simulink model "LoadControltotal2"  (R2013a)
settings: Solver=ode45  StartTime=0.0  StopTime=0.2  RelTol=1e-3
settings Model: Creator=MEHEDI HASSAN  LastModifiedBy=BORAT
settings OptimizationCC: InlineParams=on
settings DebuggingCC: SolverPrmCheckMsg=none  ModelReferenceExtraNoncontSigs=none

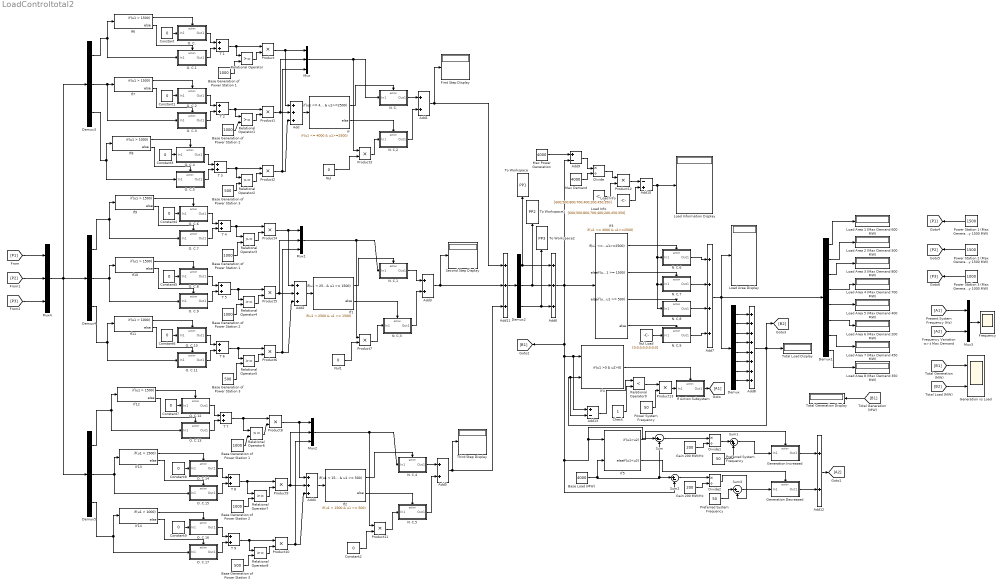
== system LoadControltotal2 ==
  Add{,2,4,6,11} (5 alike) : Sum  Inputs=+++
  Add{1,3,5,12} (4 alike) : Sum
  Add10 : Sum  Inputs=-+
  Add13 : Sum  Inputs=+-
  Add7 : Sum  Inputs=++++
  Add8 : Sum  Inputs=++++++++
  Add9 : Sum  Inputs=+-
  Base Generation of Power Station 1 : Constant  Value=1000
  "Base Generation of Power Station 1 " : Constant  Value=1000
  "Base Generation of Power Station 1  " : Constant  Value=1000
  Base Generation of Power Station 2 : Constant  Value=1000
  "Base Generation of Power Station 2 " : Constant  Value=1000
  "Base Generation of Power Station 2  " : Constant  Value=1000
  Base Generation of Power Station 3 : Constant  Value=500
  "Base Generation of Power Station 3 " : Constant  Value=500
  "Base Generation of Power Station 3  " : Constant  Value=500
  Base Load (MW) : Constant  Value=4000
  Check : Constant
  Constant{,1..9} (10 alike) : Constant  Value=0
  Demux : Demux  Outputs=8
  Demux1 : Demux  Outputs=8
  Demux{2..5} (4 alike) : Demux  Outputs=3
  Divide : Product  Inputs=*/
  Divide1 : Product  Inputs=*/
  Divide2 : Product  Inputs=*/
  First Step Display : Display
  Frequency : Scope
      settings: TickLabels=on  ShowLegends=on
  Gain 200 MW/Hz : Constant  Value=200
  "Gain 200 MW/Hz " : Constant  Value=200
  Generation Decreased : Subsystem  TreatAsAtomicUnit=on
  Generation Increased : Subsystem  TreatAsAtomicUnit=on
  Generation vs Load : Scope  NumInputPorts=2
      settings: ShowLegends=on  YMin=-5~-5  YMax=5~5
  If : If  IfExpression=u1 <= 4000 & u1>=2500
  If Action Subsystem : Subsystem  TreatAsAtomicUnit=on
  If1 : If  IfExpression=u1 < 2500 & u1 >= 1500
  If{6..7,9..10,12..13} (6 alike) : If  IfExpression=u1 > 1500
  If11 : If  IfExpression=u1 > 1000
  If14 : If  IfExpression=u1 > 1000
  If2 : If  IfExpression=u1 < 1500 & u1 >= 500
  If3 : If  IfExpression=u1 <= 4000 & u1>=2500  ElseIfExpressions=u1 < 2500 & u1 >= 1500, u1 < 1500 & u1 >= 500
  If4 : If  NumInputs=2  IfExpression=u1 >0 & u2>0  ShowElse=off
  If5 : If  NumInputs=2  IfExpression=u1>u2  ElseIfExpressions=u1<u2  ShowElse=off
  If8 : If  IfExpression=u1 > 1000
  Load Area 1 (Max Demand 600 MW) : Display
  Load Area 2 (Max Demand 500 MW) : Display
  Load Area 3 (Max Demand 800 MW) : Display
  Load Area 4 (Max Demand 700 MW) : Display
  Load Area 5 (Max Demand 400 MW) : Display
  Load Area 6 (Max Demand 200 MW) : Display
  Load Area 7 (Max Demand 450 MW) : Display
  Load Area 8 (Max Demand 350 MW) : Display
  Load Area Display : Display
  Load Info : Constant  Value=[600;500;800;700;400;200;450;350]
  "Load Info " : Constant  Value=[600;500;800;700;400;200;450;350]
  Load Information Display : Display
  Max Demand : Constant  Value=4000
  Max Power Generation : Constant  Value=4000
  Mux{,1..2,4} (4 alike) : Mux  Inputs=3
  Mux3 : Mux  Inputs=2
  N. C, : Subsystem  TreatAsAtomicUnit=on
  N. C,1 : Subsystem  TreatAsAtomicUnit=on
  N. C,2 : Subsystem  TreatAsAtomicUnit=on
  N. C,3 : Subsystem  TreatAsAtomicUnit=on
  N. C,4 : Subsystem  TreatAsAtomicUnit=on
  N. C,5 : Subsystem  TreatAsAtomicUnit=on
  N. C,6 : Subsystem  TreatAsAtomicUnit=on
  N. C,7 : Subsystem  TreatAsAtomicUnit=on
  N. C,8 : Subsystem  TreatAsAtomicUnit=on
  N. C,9 : Subsystem  TreatAsAtomicUnit=on
  Nul : Constant  Value=0
  Nul Load : Constant  Value=[0;0;0;0;0;0;0;0]
  Nul1 : Constant  Value=0
  O. C. : Subsystem  TreatAsAtomicUnit=on
  O. C.1 : Subsystem  TreatAsAtomicUnit=on
  O. C.10 : Subsystem  TreatAsAtomicUnit=on
  O. C.11 : Subsystem  TreatAsAtomicUnit=on
  O. C.12 : Subsystem  TreatAsAtomicUnit=on
  O. C.13 : Subsystem  TreatAsAtomicUnit=on
  O. C.14 : Subsystem  TreatAsAtomicUnit=on
  O. C.15 : Subsystem  TreatAsAtomicUnit=on
  O. C.16 : Subsystem  TreatAsAtomicUnit=on
  O. C.17 : Subsystem  TreatAsAtomicUnit=on
  O. C.2 : Subsystem  TreatAsAtomicUnit=on
  O. C.3 : Subsystem  TreatAsAtomicUnit=on
  O. C.4 : Subsystem  TreatAsAtomicUnit=on
  O. C.5 : Subsystem  TreatAsAtomicUnit=on
  O. C.6 : Subsystem  TreatAsAtomicUnit=on
  O. C.7 : Subsystem  TreatAsAtomicUnit=on
  O. C.8 : Subsystem  TreatAsAtomicUnit=on
  O. C.9 : Subsystem  TreatAsAtomicUnit=on
  Power Station 1 (Max Generation Capacity 1500 MW) : Constant  Value=1500
  Power Station 2 (Max Generation Capacity 1500 MW) : Constant  Value=1500
  Power Station 3 (Max Generation Capacity 1000 MW) : Constant  Value=1000
  Power System Frequency : Constant  Value=50
  Preferred System Frequency : Constant  Value=50
  "Preferred System Frequency " : Constant  Value=50
  Product{,1..13} (14 alike) : Product
  Relational Operator{,1..8} (9 alike) : RelationalOperator  OutDataTypeStr=boolean
  Relational Operator9 : RelationalOperator  Operator=<  OutDataTypeStr=boolean
  Second Step Display : Display
  Sum : Sum  Inputs=|+-
  Sum1 : Sum  Inputs=|++
  Sum2 : Sum  Inputs=|+-
  Sum3 : Sum  Inputs=|+-
  T {1..9} (9 alike) : Sum
  Third Step Display : Display
  To Workspace : ToWorkspace  VariableName=PP1  SampleTime=-1
  To Workspace1 : ToWorkspace  VariableName=PP2  SampleTime=-1
  To Workspace2 : ToWorkspace  VariableName=PP3  SampleTime=-1
  Total Generation Display : Display
  Total Load Display : Display
  wires:
  Nul Load/1 -> N. C,9/1(In1)
  If3/1 -> N. C,6/Action
  If3/2 -> N. C,7/Action
  If3/3 -> N. C,8/Action
  If3/4 -> N. C,9/Action
  Add10/1 -> Load Information Display/1, N. C,6/1(In1), N. C,7/1(In1), N. C,8/1(In1)
  N. C,6/1(Out1) -> Add7/1
  N. C,7/1(Out1) -> Add7/2
  N. C,8/1(Out1) -> Add7/3
  N. C,9/1(Out1) -> Add7/4
  Demux/1 -> Add8/1
  Demux/2 -> Add8/2
  Demux/3 -> Add8/3
  Demux/4 -> Add8/4
  Demux/5 -> Add8/5
  Demux/6 -> Add8/6
  Demux/7 -> Add8/7
  Demux/8 -> Add8/8
  Add7/1 -> Demux1/1, Load Area Display/1, Demux/1
  Add6/1 -> Add9/2, If3/1, Sum2/2, Sum/1, If5/1, Add13/1, If4/1, [B1]
  Demux2/1 -> Add6/1, To Workspace/1
  Demux2/2 -> Add6/2, To Workspace1/1
  Demux2/3 -> To Workspace2/1, Add6/3
  Max Power Generation/1 -> Add9/1
  Add9/1 -> Divide/1
  Max Demand/1 -> Divide/2
  Divide/1 -> Product12/1
  Load Info/1 -> Product12/2
  Product12/1 -> Add10/1
  "Load Info "/1 -> Add10/2
  Demux1/1 -> Load Area 1 (Max Demand 600 MW)/1
  Demux1/2 -> Load Area 2 (Max Demand 500 MW)/1
  Demux1/3 -> Load Area 3 (Max Demand 800 MW)/1
  Demux1/4 -> Load Area 4 (Max Demand 700 MW)/1
  Demux1/5 -> Load Area 5 (Max Demand 400 MW)/1
  Demux1/6 -> Load Area 6 (Max Demand 200 MW)/1
  Demux1/7 -> Load Area 7 (Max Demand 450 MW)/1
  Demux1/8 -> Load Area 8 (Max Demand 350 MW)/1
  If4/1 -> If Action Subsystem/Action
  Add8/1 -> [B2], Total Load Display/1, Add13/2, If4/2
  Sum/1 -> Divide1/1
  Gain 200 MW/Hz/1 -> Divide1/2
  Divide1/1 -> Sum1/1
  Preferred System Frequency/1 -> Sum1/2
  Sum1/1 -> Generation Increased/1(In1)
  Base Load (MW)/1 -> Sum2/1, Sum/2, If5/2
  Sum2/1 -> Divide2/1
  "Gain 200 MW/Hz "/1 -> Divide2/2
  Divide2/1 -> Sum3/2
  "Preferred System Frequency "/1 -> Sum3/1
  Sum3/1 -> Generation Decreased/1(In1)
  If5/1 -> Generation Increased/Action
  If5/2 -> Generation Decreased/Action
  Generation Increased/1(Out1) -> Add12/1
  Generation Decreased/1(Out1) -> Add12/2
  Mux3/1 -> Frequency/1
  [B1] -> Generation vs Load/1
  [B2] -> Generation vs Load/2
  [A1] -> Mux3/1
  [A2] -> Mux3/2
  If Action Subsystem/1(Out1) -> [A1]
  Add12/1 -> [A2]
  Power Station 1 (Max Generation Capacity 1500 MW)/1 -> [P1]
  Power Station 2 (Max Generation Capacity 1500 MW)/1 -> [P2]
  Power Station 3 (Max Generation Capacity 1000 MW)/1 -> [P3]
  [B1] -> Total Generation Display/1
  Check/1 -> Relational Operator9/2
  Relational Operator9/1 -> Product13/1
  Power System Frequency/1 -> Product13/2
  Add13/1 -> Relational Operator9/1
  Product13/1 -> If Action Subsystem/1(In1)
  Base Generation of Power Station 1/1 -> Relational Operator/2
  Relational Operator/1 -> Product/2
  Base Generation of Power Station 2/1 -> Relational Operator1/2
  Relational Operator1/1 -> Product1/2
  Base Generation of Power Station 3/1 -> Relational Operator2/2
  Relational Operator2/1 -> Product2/2
  Product/1 -> Mux/1, Add/1
  Product1/1 -> Add/2, Mux/2
  Product2/1 -> Add/3, Mux/3
  Add/1 -> If/1
  If/2 -> N. C,2/Action
  Mux/1 -> N. C,/1(In1), Product3/1
  Product3/1 -> N. C,2/1(In1)
  Nul/1 -> Product3/2
  N. C,/1(Out1) -> Add1/1
  If/1 -> N. C,/Action
  Add1/1 -> Add11/1, First Step Display/1
  N. C,2/1(Out1) -> Add1/2
  "Base Generation of Power Station 1 "/1 -> Relational Operator3/2
  Relational Operator3/1 -> Product4/2
  "Base Generation of Power Station 2 "/1 -> Relational Operator4/2
  Relational Operator4/1 -> Product5/2
  "Base Generation of Power Station 3 "/1 -> Relational Operator5/2
  Relational Operator5/1 -> Product6/2
  Product4/1 -> Mux1/1, Add2/1
  Product5/1 -> Add2/2, Mux1/2
  Product6/1 -> Add2/3, Mux1/3
  Add2/1 -> If1/1
  If1/1 -> N. C,1/Action
  If1/2 -> N. C,3/Action
  Mux1/1 -> Product7/1, N. C,1/1(In1)
  Product7/1 -> N. C,3/1(In1)
  Nul1/1 -> Product7/2
  N. C,1/1(Out1) -> Add3/1
  Add3/1 -> Add11/2, Second Step Display/1
  N. C,3/1(Out1) -> Add3/2
  "Base Generation of Power Station 1  "/1 -> Relational Operator6/2
  Relational Operator6/1 -> Product8/2
  "Base Generation of Power Station 2  "/1 -> Relational Operator7/2
  Relational Operator7/1 -> Product9/2
  "Base Generation of Power Station 3  "/1 -> Relational Operator8/2
  Relational Operator8/1 -> Product10/2
  Product8/1 -> Mux2/1, Add4/1
  Product9/1 -> Add4/2, Mux2/2
  Product10/1 -> Add4/3, Mux2/3
  Add4/1 -> If2/1
  If2/1 -> N. C,4/Action
  If2/2 -> N. C,5/Action
  Mux2/1 -> N. C,4/1(In1), Product11/1
  Product11/1 -> N. C,5/1(In1)
  Constant2/1 -> Product11/2
  N. C,4/1(Out1) -> Add5/1
  N. C,5/1(Out1) -> Add5/2
  Add5/1 -> Add11/3, Third Step Display/1
  Add11/1 -> Demux2/1
  [P1] -> Mux4/1
  [P2] -> Mux4/2
  [P3] -> Mux4/3
  Constant/1 -> O. C./1(In1)
  Demux3/1 -> O. C.1/1(In1), If6/1
  If6/1 -> O. C./Action
  If6/2 -> O. C.1/Action
  O. C./1(Out1) -> T 1/1
  O. C.1/1(Out1) -> T 1/2
  T 1/1 -> Product/1, Relational Operator/1
  Constant1/1 -> O. C.2/1(In1)
  Demux3/2 -> O. C.3/1(In1), If7/1
  If7/1 -> O. C.2/Action
  If7/2 -> O. C.3/Action
  O. C.2/1(Out1) -> T 2/1
  O. C.3/1(Out1) -> T 2/2
  T 2/1 -> Relational Operator1/1, Product1/1
  Constant3/1 -> O. C.4/1(In1)
  Demux3/3 -> If8/1, O. C.5/1(In1)
  If8/1 -> O. C.4/Action
  If8/2 -> O. C.5/Action
  O. C.4/1(Out1) -> T 3/1
  O. C.5/1(Out1) -> T 3/2
  T 3/1 -> Product2/1, Relational Operator2/1
  Constant4/1 -> O. C.6/1(In1)
  Demux4/1 -> O. C.7/1(In1), If9/1
  If9/1 -> O. C.6/Action
  If9/2 -> O. C.7/Action
  O. C.6/1(Out1) -> T 4/1
  O. C.7/1(Out1) -> T 4/2
  T 4/1 -> Product4/1, Relational Operator3/1
  Constant5/1 -> O. C.8/1(In1)
  Demux4/2 -> O. C.9/1(In1), If10/1
  If10/1 -> O. C.8/Action
  If10/2 -> O. C.9/Action
  O. C.8/1(Out1) -> T 5/1
  O. C.9/1(Out1) -> T 5/2
  T 5/1 -> Product5/1, Relational Operator4/1
  Constant6/1 -> O. C.10/1(In1)
  Demux4/3 -> If11/1, O. C.11/1(In1)
  If11/1 -> O. C.10/Action
  If11/2 -> O. C.11/Action
  O. C.10/1(Out1) -> T 6/1
  O. C.11/1(Out1) -> T 6/2
  T 6/1 -> Product6/1, Relational Operator5/1
  Constant7/1 -> O. C.12/1(In1)
  Demux5/1 -> O. C.13/1(In1), If12/1
  If12/1 -> O. C.12/Action
  If12/2 -> O. C.13/Action
  O. C.12/1(Out1) -> T 7/1
  O. C.13/1(Out1) -> T 7/2
  T 7/1 -> Relational Operator6/1, Product8/1
  Constant8/1 -> O. C.14/1(In1)
  Demux5/2 -> O. C.15/1(In1), If13/1
  If13/1 -> O. C.14/Action
  If13/2 -> O. C.15/Action
  O. C.14/1(Out1) -> T 8/1
  O. C.15/1(Out1) -> T 8/2
  T 8/1 -> Relational Operator7/1, Product9/1
  Constant9/1 -> O. C.16/1(In1)
  Demux5/3 -> If14/1, O. C.17/1(In1)
  If14/1 -> O. C.16/Action
  If14/2 -> O. C.17/Action
  O. C.16/1(Out1) -> T 9/1
  O. C.17/1(Out1) -> T 9/2
  T 9/1 -> Relational Operator8/1, Product10/1
  Mux4/1 -> Demux5/1, Demux3/1, Demux4/1

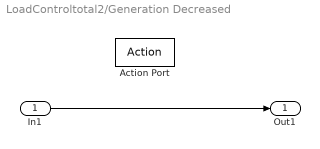
== system LoadControltotal2/Generation Decreased ==
  In1 : Inport
  Action Port : ActionPort  ActionType=elseif
  Out1 : Outport
  wires:
  In1/1 -> Out1/1

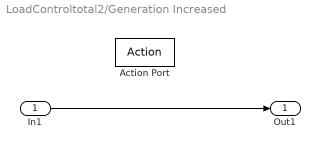
== system LoadControltotal2/Generation Increased ==
  In1 : Inport
  Action Port : ActionPort  ActionType=then
  Out1 : Outport
  wires:
  In1/1 -> Out1/1

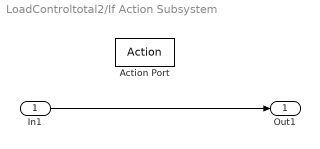
== system LoadControltotal2/If Action Subsystem ==
  In1 : Inport
  Action Port : ActionPort  ActionType=then
  Out1 : Outport
  wires:
  In1/1 -> Out1/1

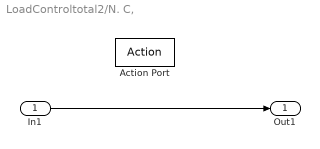
== system LoadControltotal2/N. C, ==
  In1 : Inport
  Action Port : ActionPort  ActionType=then
  Out1 : Outport
  wires:
  In1/1 -> Out1/1

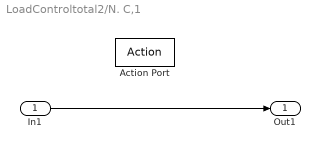
== system LoadControltotal2/N. C,1 ==
  In1 : Inport
  Action Port : ActionPort  ActionType=then
  Out1 : Outport
  wires:
  In1/1 -> Out1/1

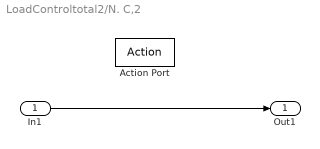
== system LoadControltotal2/N. C,2 ==
  In1 : Inport
  Action Port : ActionPort  ActionType=else
  Out1 : Outport
  wires:
  In1/1 -> Out1/1

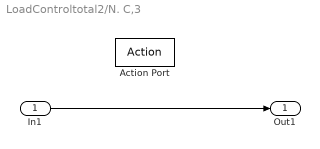
== system LoadControltotal2/N. C,3 ==
  In1 : Inport
  Action Port : ActionPort  ActionType=else
  Out1 : Outport
  wires:
  In1/1 -> Out1/1

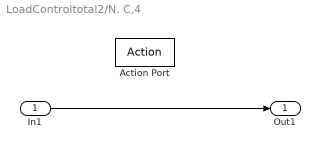
== system LoadControltotal2/N. C,4 ==
  In1 : Inport
  Action Port : ActionPort  ActionType=then
  Out1 : Outport
  wires:
  In1/1 -> Out1/1

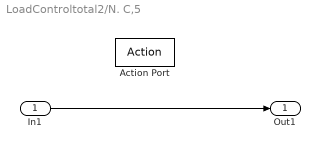
== system LoadControltotal2/N. C,5 ==
  In1 : Inport
  Action Port : ActionPort  ActionType=else
  Out1 : Outport
  wires:
  In1/1 -> Out1/1

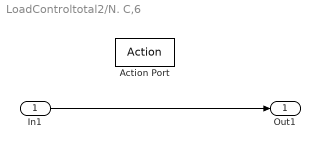
== system LoadControltotal2/N. C,6 ==
  In1 : Inport
  Action Port : ActionPort  ActionType=then
  Out1 : Outport
  wires:
  In1/1 -> Out1/1

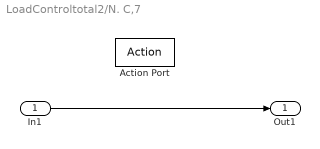
== system LoadControltotal2/N. C,7 ==
  In1 : Inport
  Action Port : ActionPort  ActionType=elseif
  Out1 : Outport
  wires:
  In1/1 -> Out1/1

== system LoadControltotal2/N. C,8 ==
  In1 : Inport
  Action Port : ActionPort  ActionType=elseif
  Out1 : Outport
  wires:
  In1/1 -> Out1/1

== system LoadControltotal2/N. C,9 ==
  In1 : Inport
  Action Port : ActionPort  ActionType=else
  Out1 : Outport
  wires:
  In1/1 -> Out1/1

== system LoadControltotal2/O. C. ==
  In1 : Inport
  Action Port : ActionPort  ActionType=then
  Out1 : Outport
  wires:
  In1/1 -> Out1/1

== system LoadControltotal2/O. C.1 ==
  In1 : Inport
  Action Port : ActionPort  ActionType=else
  Out1 : Outport
  wires:
  In1/1 -> Out1/1

== system LoadControltotal2/O. C.10 ==
  In1 : Inport
  Action Port : ActionPort  ActionType=then
  Out1 : Outport
  wires:
  In1/1 -> Out1/1

== system LoadControltotal2/O. C.11 ==
  In1 : Inport
  Action Port : ActionPort  ActionType=else
  Out1 : Outport
  wires:
  In1/1 -> Out1/1

== system LoadControltotal2/O. C.12 ==
  In1 : Inport
  Action Port : ActionPort  ActionType=then
  Out1 : Outport
  wires:
  In1/1 -> Out1/1

== system LoadControltotal2/O. C.13 ==
  In1 : Inport
  Action Port : ActionPort  ActionType=else
  Out1 : Outport
  wires:
  In1/1 -> Out1/1

== system LoadControltotal2/O. C.14 ==
  In1 : Inport
  Action Port : ActionPort  ActionType=then
  Out1 : Outport
  wires:
  In1/1 -> Out1/1

== system LoadControltotal2/O. C.15 ==
  In1 : Inport
  Action Port : ActionPort  ActionType=else
  Out1 : Outport
  wires:
  In1/1 -> Out1/1

== system LoadControltotal2/O. C.16 ==
  In1 : Inport
  Action Port : ActionPort  ActionType=then
  Out1 : Outport
  wires:
  In1/1 -> Out1/1

== system LoadControltotal2/O. C.17 ==
  In1 : Inport
  Action Port : ActionPort  ActionType=else
  Out1 : Outport
  wires:
  In1/1 -> Out1/1

== system LoadControltotal2/O. C.2 ==
  In1 : Inport
  Action Port : ActionPort  ActionType=then
  Out1 : Outport
  wires:
  In1/1 -> Out1/1

== system LoadControltotal2/O. C.3 ==
  In1 : Inport
  Action Port : ActionPort  ActionType=else
  Out1 : Outport
  wires:
  In1/1 -> Out1/1

== system LoadControltotal2/O. C.4 ==
  In1 : Inport
  Action Port : ActionPort  ActionType=then
  Out1 : Outport
  wires:
  In1/1 -> Out1/1

== system LoadControltotal2/O. C.5 ==
  In1 : Inport
  Action Port : ActionPort  ActionType=else
  Out1 : Outport
  wires:
  In1/1 -> Out1/1

== system LoadControltotal2/O. C.6 ==
  In1 : Inport
  Action Port : ActionPort  ActionType=then
  Out1 : Outport
  wires:
  In1/1 -> Out1/1

== system LoadControltotal2/O. C.7 ==
  In1 : Inport
  Action Port : ActionPort  ActionType=else
  Out1 : Outport
  wires:
  In1/1 -> Out1/1

== system LoadControltotal2/O. C.8 ==
  In1 : Inport
  Action Port : ActionPort  ActionType=then
  Out1 : Outport
  wires:
  In1/1 -> Out1/1

== system LoadControltotal2/O. C.9 ==
  In1 : Inport
  Action Port : ActionPort  ActionType=else
  Out1 : Outport
  wires:
  In1/1 -> Out1/1
